simulink model "example_SolarCollector1xN_comparison"  (R2018b)
settings: Solver=ode45  StartTime=0.0  StopTime=2*24*3600  MaxStep=1800  RelTol=1e-3  EnableMultiTasking=on
libraries: carnot x11
settings Model: Creator=drhf  LastModifiedBy=drhf
settings DataIOCC: LimitDataPoints=on  SaveFormat=Array
settings OptimizationCC: ExpressionDepthLimit=2147483647  LifeSpan=inf
settings DebuggingCC: UnderspecifiedInitializationDetection=Classic  MergeDetectMultiDrivingBlocksExec=none  SolverPrmCheckMsg=warning  StateNameClashWarn=warning  SFUnexpectedBacktrackingDiag=warning  SFNoUnconditionalDefaultTransitionDiag=warning  SFExecutionAtInitializationDiag=none
settings HardwareCC: ProdBitPerPointer=32  ProdBitPerSizeT=32  ProdBitPerPtrDiffT=32  ProdLargestAtomicFloat=None  ProdIntDivRoundTo=Undefined  ProdEndianess=Unspecified  ProdWordSize=32  ProdHWDeviceType=32-bit Generic
settings ModelReferenceCC: PropagateSignalLabelsOutOfModel=off
settings SFSimCC: SimUseLocalCustomCode=off
settings RTWCC: RTWUseLocalCustomCode=off
settings CodeAppCC: StateflowObjectComments=on
settings GRTTargetCC: TargetLangStandard=C89/C90 (ANSI)  GeneratePreprocessorConditionals=Disable all  CombineOutputUpdateFcns=off  GRTInterface=on
settings ConfigComp: CovMetricSettings=dw  CovHtmlReporting=on  CovSaveCumulativeToWorkspaceVar=on  CovSaveSingleToWorkspaceVar=on  CovExternalEMLEnable=off

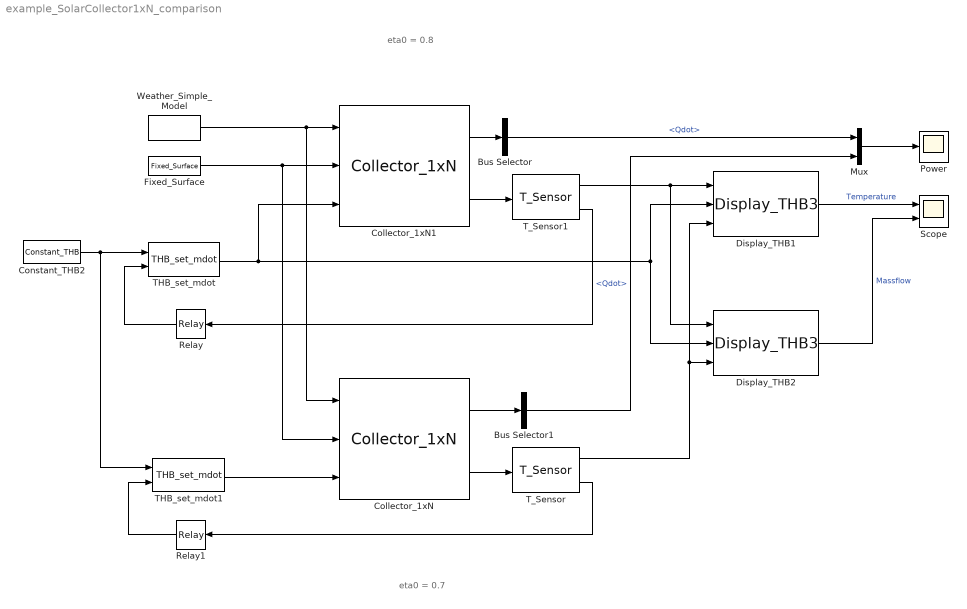
== system example_SolarCollector1xN_comparison ==
  note: eta0 = 0.7
  note: eta0 = 0.8
  Bus Selector : BusSelector  OutputSignals=Qdot
  Bus Selector1 : BusSelector  OutputSignals=Qdot
  Collector_1xN : carnot/Source/Solar_Thermal/Collector_1xN  acol=2.3  len=2  eta0=0.7  u1=3.5  u2=0.02  u3=0  uwind=0  c_col=1e4  lin=10  qua=10  tini=20  nodes=5
      settings: SourceProductName=Carnot
  Collector_1xN1 : carnot/Source/Solar_Thermal/Collector_1xN  acol=2.3  len=2  eta0=0.8  u1=3.5  u2=0.02  u3=0  uwind=0  c_col=1e4  lin=10  qua=10  tini=20  nodes=5
      settings: SourceProductName=Carnot
  Constant_THB2 : carnot/Source/Simple/Constant_THB  t=40  mdot=100/3600  p=1e5  mID=No Pressure Drop  fluid=Water  mix=0  mix2=0  mix3=0  dia=0.02  hgt=0
      settings: SourceProductName=Carnot
  Display_THB1 : carnot/Outputs/Display_THB3  t=on  m=off  p=off  id=off  mix=off  d=off
      settings: SourceProductName=Carnot
  Display_THB2 : carnot/Outputs/Display_THB3  t=off  m=on  p=off  id=off  mix=off  d=off
      settings: SourceProductName=Carnot
  Fixed_Surface : carnot/Weather/Fixed_Surface  colangle=30  colazi=0  colrot=0
      settings: SourceProductName=Carnot
  Mux : Mux  Inputs=2
  Power : Scope
  Relay : Relay  OnSwitchValue=47  OffSwitchValue=42  OnOutputValue=50/3600
  Relay1 : Relay  OnSwitchValue=47  OffSwitchValue=42  OnOutputValue=50/3600
  Scope : Scope  NumInputPorts=2
  THB_set_mdot : carnot/Source/Simple/THB_set_mdot
      settings: SourceProductName=Carnot
  THB_set_mdot1 : carnot/Source/Simple/THB_set_mdot
      settings: SourceProductName=Carnot
  T_Sensor : carnot/Control/T_Sensor  tc=10  t0=20
      settings: SourceProductName=Carnot
  T_Sensor1 : carnot/Control/T_Sensor  tc=10  t0=20
      settings: SourceProductName=Carnot
  Weather_Simple_Model : carnot/Weather/Weather_Simple_Model  lat=60  Ibn=900  Idg=100  tamb=5  deltaTsky=-6  rh=50  precip="10e-3/24/3600           % 10 mm in 24 h"  cloud=0.125  p=1013e2  vw=1  wdir=270
      settings: SourceProductName=Carnot
  wires:
  Weather_Simple_Model/1 -> Collector_1xN1/1, Collector_1xN/1
  Fixed_Surface/1 -> Collector_1xN1/2, Collector_1xN/2
  THB_set_mdot/1 -> Collector_1xN1/3, Display_THB1/2, Display_THB2/2
  Display_THB1/1 -> Scope/1  "Temperature"
  Collector_1xN1/1 -> Bus Selector/1
  Bus Selector/1 -> Mux/1  "<Qdot>"
  Bus Selector1/1 -> Mux/2  "<Qdot>"
  Mux/1 -> Power/1
  Constant_THB2/1 -> THB_set_mdot/1, THB_set_mdot1/1
  THB_set_mdot1/1 -> Collector_1xN/3
  T_Sensor/1 -> Display_THB1/3, Display_THB2/3
  Relay/1 -> THB_set_mdot/2
  T_Sensor/2 -> Relay1/1
  Relay1/1 -> THB_set_mdot1/2
  T_Sensor1/1 -> Display_THB1/1, Display_THB2/1
  Display_THB2/1 -> Scope/2  "Massflow"
  Collector_1xN/1 -> Bus Selector1/1
  Collector_1xN/2 -> T_Sensor/1
  Collector_1xN1/2 -> T_Sensor1/1
  T_Sensor1/2 -> Relay/1
